simulink model "test_SET_IET_Blocks"  (Simulink 4.00)
settings: Solver=FixedStepDiscrete  StartTime=0.0  StopTime=60  FixedStep=0.05  RelTol=1e-3
libraries: simulink3 x4
settings Model: LastModifiedBy=bsaunder

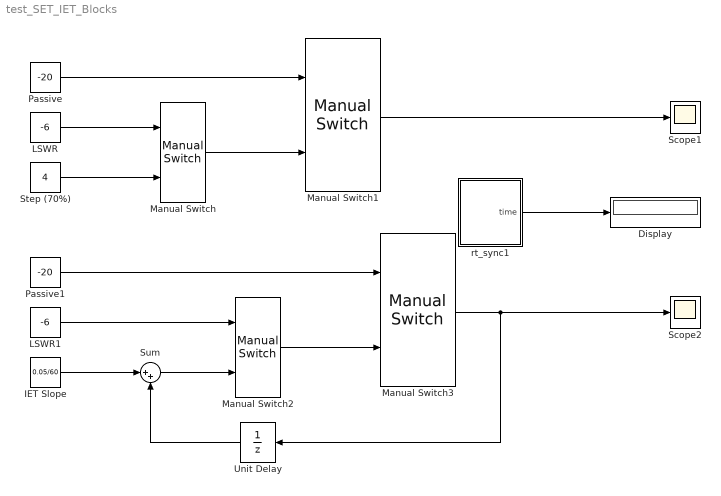
== system test_SET_IET_Blocks ==
  Display : Display
      settings: Format=short
  IET Slope : Constant  Value=0.05/60
  LSWR : Constant  Value=-6
  LSWR1 : Constant  Value=-6
  Manual Switch{,1..3} (4 alike) : simulink3/Nonlinear/Manual Switch  sw=1  action=0
  Passive : Constant  Value=-20
  Passive1 : Constant  Value=-20
  Scope1 : Scope
      settings: TimeRange=60  YMin=-20  YMax=-20  SaveToWorkspace=off  LimitDataPoints=on  MaxDataPoints=5000
  Scope2 : Scope
      settings: TimeRange=60  YMin=-8.67362e-019  YMax=0.0325  SaveToWorkspace=off  SaveName=ScopeData  LimitDataPoints=on  MaxDataPoints=5000
  Step (70%) : Constant  Value=4
  Sum : Sum  Inputs=|++  SaturateOnIntegerOverflow=on
  Unit Delay : UnitDelay  Orientation=left  X0=-20  SampleTime=-1
      settings: RTWStateStorageClass=Auto
  rt_sync1 : Subsystem  mask{Ts=0.05}
      mask prompts: Ts "Sample Time"
      settings: RTWFcnNameOpts=Auto  RTWFileNameOpts=Auto
      mask Display: fprintf('Real\n Time\n sync')
  wires:
  Manual Switch/1 -> Manual Switch1/2
  Step (70%)/1 -> Manual Switch/2
  LSWR/1 -> Manual Switch/1
  Passive/1 -> Manual Switch1/1
  Manual Switch1/1 -> Scope1/1
  Manual Switch2/1 -> Manual Switch3/2
  LSWR1/1 -> Manual Switch2/1
  Passive1/1 -> Manual Switch3/1
  IET Slope/1 -> Sum/1
  Sum/1 -> Manual Switch2/2
  Unit Delay/1 -> Sum/2
  Manual Switch3/1 -> Unit Delay/1, Scope2/1
  rt_sync1/1(time) -> Display/1

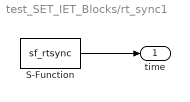
== system test_SET_IET_Blocks/rt_sync1 ==
  S-Function : S-Function  FunctionName=sf_rtsync  Parameters=Ts  PortCounts=[]  SFunctionModules=''
  time : Outport  Port=1
  wires:
  S-Function/1 -> time/1
